simulink model "speedgoat_IO397_TPI6020"  (R2023a)
settings: Solver=FixedStepDiscrete  StartTime=0.0  StopTime=inf  RelTol=1e-3
PreLoadFcn:
  | if ~exist('Ts', 'var')
  | Ts = 0.001;
  | end
  | if ~exist('FPGA_Frequency', 'var')
  | FPGA_Frequency = 75000000;
  | end
  | if ~exist('Tpwm', 'var')
  | Tpwm = 0.005;
  | end
undefined symbols (not defined in the file): IO397
libraries: speedgoatlib_fpga_dio x2, speedgoatlib_fpga_analog_io x2, speedgoatlib_fpga_pwm x1, speedgoatlib_fpga_quadrature x1, speedgoatlib_fpga x1
settings Model: Creator=simon.beck  LastModifiedBy=jeffrey.gruenig
settings SolverCC: ConcurrentTasks=on  PositivePriorityOrder=on
settings DataIOCC: SaveFormat=StructureWithTime
settings OptimizationCC: BlockReduction=off  OptimizeBlockIOStorage=off  BufferReuse=off
settings DebuggingCC: UnderspecifiedInitializationDetection=Classic  MergeDetectMultiDrivingBlocksExec=none  TasksWithSamePriorityMsg=none
settings HardwareCC: ProdBitPerLong=64  ProdLongLongMode=on  ProdHWDeviceType=Intel->x86-64 (Linux 64)
settings ModelReferenceCC: EnableRefExpFcnMdlSchedulingChecks=on  PropagateSignalLabelsOutOfModel=off
settings RTWCC: Description=Simulink Real-Time  SystemTargetFile=slrealtime.tlc  TemplateMakefile=slrealtime_default_tmf  Toolchain=Simulink Real-Time Toolchain  BuildConfiguration=Faster Runs  CodeExecutionProfiling=on  TargetLang=C++  DLArmComputeVersion=19.05

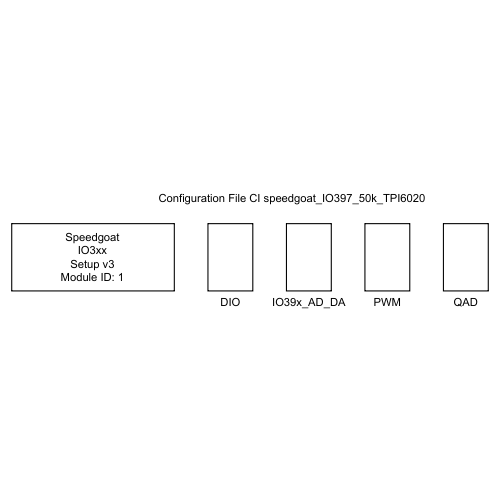
[thumbnail: Simulink's stored preview of the top-level diagram]
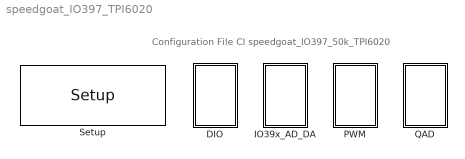
== system speedgoat_IO397_TPI6020 ==
  note: Configuration File CI speedgoat_IO397_50k_TPI6020
  DIO : Subsystem
  IO39x_AD_DA : Subsystem
  PWM : Subsystem
  QAD : Subsystem
  Setup : speedgoatlib_fpga/Setup/Setup  board=IO397-50k  id=1  device_id=1  frontIO=None  rearIO=None  bitstreamFile=speedgoat_IO397_TPI6020.mat  rev=6.100000  timestamp_string=06/12/23 16:33:50  fpgaFreq=75 MHz  fpgaTick=13.33 ns  ProgSpiFlash=off  ProgBPIFlash=off  pciSlot=-1  useFpgaDmaController=off  PullRPort0=pull-up 3.3V  VioPort0=3.3V  PullRPort1=pull-up 3.3V  VioPort1=3.3V  PullRPort2=pull-up 3.3V  VioPort2=3.3V  PullRPort3=pull-up 3.3V  VioPort3=3.3V  PullRPort4=pull-up 3.3V  VioPort4=3.3V  PullRPort5=pull-up 3.3V  VioPort5=3.3V  PullRPort6=pull-up 3.3V  VioPort6=3.3V  diffLineTermination_rear1=on  diffLineTermination_rear2=on  diffLineTermination_rear3=on  diffLineTermination_rear4=on  diffLineTermination_rear5=on  diffLineTermination_rear6=on  diffLineTermination_rear7=on  diffLineTermination_rear8=on  PullRPort15=pull-up 3.3V  PullRPort31=pull-up 3.3V  PullRPort47=pull-up 3.3V  PullRPort63=pull-up 3.3V  diffLineTermination_1=on  diffLineTermination_2=on  diffLineTermination_3=on  diffLineTermination_4=on  diffLineTermination_5=on  diffLineTermination_6=on  diffLineTermination_7=on  diffLineTermination_8=on  diffLineTermination_9=on  diffLineTermination_10=on  diffLineTermination_11=on  diffLineTermination_12=on  diffLineTermination_13=on  diffLineTermination_14=on  diffLineTermination_15=on  diffLineTermination_16=on  diffLineTermination_17=on  diffLineTermination_18=on  diffLineTermination_19=on  diffLineTermination_20=on  diffLineTermination_21=on  diffLineTermination_22=on  diffLineTermination_23=on  diffLineTermination_24=on  diffLineTermination_25=on  diffLineTermination_26=on  diffLineTermination_27=on  diffLineTermination_28=on  diffLineTermination_29=on  diffLineTermination_30=on  diffLineTermination_31=on  diffLineTermination_32=on  Vo_36x_1=3.3V  Vi_Pull_36x_1=Floating  Vo_36x_2=3.3V  Vi_Pull_36x_2=Floating  Vo_36x_3=3.3V  Vi_Pull_36x_3=Floating  Vo_36x_4=3.3V  Vi_Pull_36x_4=Floating  Vo_36x_5=3.3V  Vi_Pull_36x_5=Floating  Vo_36x_6=3.3V  Vi_Pull_36x_6=Floating  Vo_36x_7=3.3V  Vi_Pull_36x_7=Floating  Vo_36x_8=3.3V  Vi_Pull_36x_8=Floating  Vo_36x_9_16=3.3V  Vi_Pull_36x_9_16=Floating  Vo_36x_17_24=3.3V  Vi_Pull_36x_17_24=Floating  Vo_36x_25_32=3.3V  Vi_Pull_36x_25_32=Floating  Vo_36x_33_40=3.3V  Vi_Pull_36x_33_40=Floating  Vo_36x_41_48=3.3V  Vi_Pull_36x_41_48=Floating  Vo_36x_49_56=3.3V  Vi_Pull_36x_49_56=Floating  Vo_36x_57_64=3.3V  Vi_Pull_36x_57_64=Floating
      settings: SourceProductName=Simulink Real-Time: Speedgoat I/O Blockset

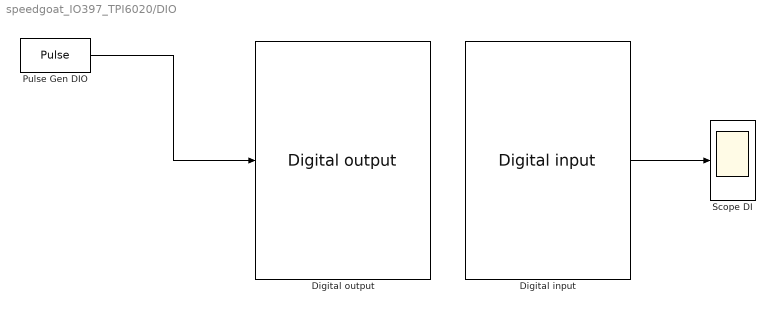
== system speedgoat_IO397_TPI6020/DIO ==
  Digital input : speedgoatlib_fpga_dio/Digital input  id=1  chan=[14]  ts=Ts  vectorizeOutput=on
      settings: SourceProductName=Simulink Real-Time: Speedgoat I/O Blockset
  Digital output : speedgoatlib_fpga_dio/Digital output  id=1  chan=[13]  init=[0]  reset=[0]  ts=Ts  vectorizeInput=off
      settings: SourceProductName=Simulink Real-Time: Speedgoat I/O Blockset
  Pulse Gen DIO : DiscretePulseGenerator  Period=20  PulseWidth=10  SampleTime=Ts  VectorParams1D=off
  Scope DI : Scope
  wires:
  Digital input/1 -> Scope DI/1
  Pulse Gen DIO/1 -> Digital output/1

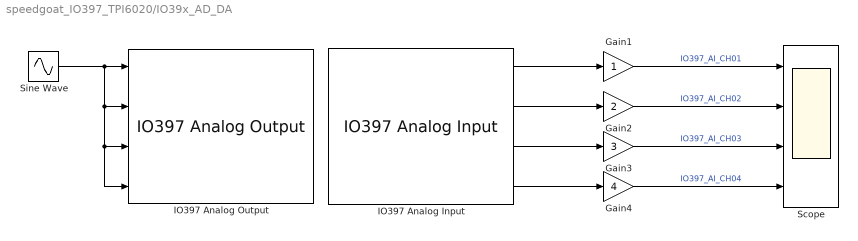
== system speedgoat_IO397_TPI6020/IO39x_AD_DA ==
  Gain1 : Gain
  Gain2 : Gain  Gain=2
  Gain3 : Gain  Gain=3
  Gain4 : Gain  Gain=4
  IO397 Analog Input : speedgoatlib_fpga_analog_io/IO397 Analog Input  openMaskCallback=0  id=1  chan=[1:4]  range=+-5 V  parAiTriggerMode=I/O Module Clock  parAiInternalSignal=None  parAiDioTriggerChannel=13  parAiSampleRate=0  trigger=Initiator  ts=0.001
      settings: SourceProductName=Simulink Real-Time: Speedgoat I/O Blockset
  IO397 Analog Output : speedgoatlib_fpga_analog_io/IO397 Analog Output  id=1  chan=1:4  initVal=0  resetVal=0  ts=0.001  span=+-5 V
      settings: SourceProductName=Simulink Real-Time: Speedgoat I/O Blockset
  Scope : Scope  NumInputPorts=4
  Sine Wave : Sin  Frequency=2*pi*(1/Ts)/50  SampleTime=Ts
  wires:
  IO397 Analog Input/4 -> Gain4/1
  IO397 Analog Input/3 -> Gain3/1
  IO397 Analog Input/2 -> Gain2/1
  IO397 Analog Input/1 -> Gain1/1
  Gain4/1 -> Scope/4  "IO397_AI_CH04"
  Gain3/1 -> Scope/3  "IO397_AI_CH03"
  Gain2/1 -> Scope/2  "IO397_AI_CH02"
  Gain1/1 -> Scope/1  "IO397_AI_CH01"
  Sine Wave/1 -> IO397 Analog Output/1, IO397 Analog Output/3, IO397 Analog Output/4, IO397 Analog Output/2

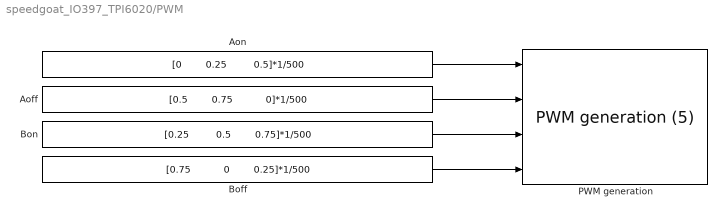
== system speedgoat_IO397_TPI6020/PWM ==
  Aoff : Constant  Value="[0.5        0.75           0]*1/500"  OutDataTypeStr=Inherit: Inherit via back propagation  SampleTime=-1
  Aon : Constant  Value="[0        0.25         0.5]*1/500"  VectorParams1D=off  OutDataTypeStr=Inherit: Inherit via back propagation  SampleTime=-1
  Boff : Constant  Value="[0.75           0        0.25]*1/500"  OutDataTypeStr=Inherit: Inherit via back propagation  SampleTime=-1
  Bon : Constant  Value="[0.25         0.5        0.75]*1/500"  OutDataTypeStr=Inherit: Inherit via back propagation  SampleTime=-1
  PWM generation : speedgoatlib_fpga_pwm/PWM generation (5)  id=1  chan=[1:3]  board=IO397-50k  ts=0.001  enableDma=off  pciSlot=[-1,-1]  delay=0  symmetric=Asymmetric - On and Off are freely configurable  b_is_complement_of_a=Independent of PWM A output  deadband=[0.0]  period=[1/500]  frequency=500  ticks=149999  a_on=0  a_off=0.5e-3  pwm_a_dc=[0.0]  b_on=0.25e-3  b_off=0.75e-3  pwm_b_dc=[0]  c_on=[0.0]  c_off=[0.0]  protection=Disabled: A and B can be high at the same moment  enable_latch_half_period=off  pwm_update=At period starts  bit_width_pwm_gen=24  trigger_duration=[10e-6]  trigger_period_start=on  trigger_half_of_the_period=off  trigger_a_on=off  trigger_a_off=off  trigger_b_on=off  trigger_b_off=off  show_a_input=on  show_b_input=on  show_c_input=off  show_period_input=off  show_force_stop_input=off  idle_a=Low when PWM generation is halted  idle_b=Low when PWM generation is halted  idle_c=Low when PWM generation is halted  cancels_pwm_generation=on  invert_a=off  invert_b=off  invert_c=off
      settings: SourceProductName=Simulink Real-Time: Speedgoat I/O Blockset
  wires:
  Boff/1 -> PWM generation/4
  Bon/1 -> PWM generation/3
  Aoff/1 -> PWM generation/2
  Aon/1 -> PWM generation/1

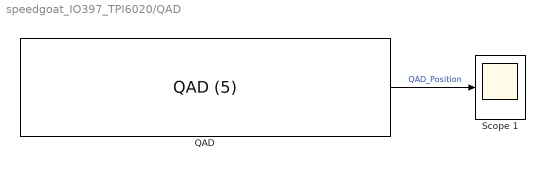
== system speedgoat_IO397_TPI6020/QAD ==
  QAD : speedgoatlib_fpga_quadrature/QAD (5)  id=1  chan=[1:1]  sampleTime=0.001  enableDma=on  numOfSlots=[16]  sensorType=Capture A + B Signal  interpolatePosition=off  swapAB=off  indexControlMode=Ignore Index  latchMode=Disabled  gateIndex=No Gating  speedFilterWidth=4  showInputSpeedFilterWidth=off  glitchFilterSeconds=106.7e-9  glitchFilterSecondsEff=106.7e-9  showInputClearPosition=off  showInputClearIndexFound=off  showOutputPosition=on  showOutputTurn=off  showOutputSpeed=off  showOutputIndexFound=off  showOutputLastPulse=off
      settings: SourceProductName=Simulink Real-Time: Speedgoat I/O Blockset
  "Scope 1 " : Scope
  wires:
  QAD/1 -> "Scope 1 "/1  "QAD_Position"
